simulink model "PMSM_RobotKinematics"  (R2018b)
settings: Solver=VariableStepAuto  StartTime=0.0  StopTime=0.2  FixedStep=Ts  RelTol=1e-4  EnableMultiTasking=on
PreLoadFcn:
  | run('Arm6Assembly_DataFile.m');
model workspace: external: MAT-File E:\SixRobotArm\Simscape_Simulation\StepFile\Arm6Assembly_DataFile.mat (data not in the file)
values from neighbouring files (symbols this model uses):
  smiData =     [Arm6SimscapeData.mat]
undefined symbols (not defined in the file or in its folder): X, Y, Z
libraries: sm_lib x36, fl_lib x25, nesl_utility x19, simulink_extras x7
(part 1 of 4)
settings Model: Creator=SUN  LastModifiedBy=Jeason
settings SolverCC: ZeroCrossControl=DisableAll
settings DataIOCC: LimitDataPoints=on  SaveFormat=Array  SignalLoggingSaveFormat=ModelDataLogs
settings OptimizationCC: ExpressionDepthLimit=2147483647  InitFltsAndDblsToZero=on  LifeSpan=inf
settings DebuggingCC: UnderspecifiedInitializationDetection=Classic  MergeDetectMultiDrivingBlocksExec=none  SolverPrmCheckMsg=warning  FcnCallInpInsideContextMsg=warning  StateNameClashWarn=warning  SFUnexpectedBacktrackingDiag=warning  SFNoUnconditionalDefaultTransitionDiag=warning  SFExecutionAtInitializationDiag=none
settings HardwareCC: ProdBitPerPointer=32  ProdBitPerSizeT=32  ProdBitPerPtrDiffT=32  ProdLargestAtomicFloat=None  ProdIntDivRoundTo=Undefined  ProdEndianess=Unspecified  ProdWordSize=32  ProdHWDeviceType=32-bit Generic
settings ModelReferenceCC: PropagateSignalLabelsOutOfModel=off
settings SFSimCC: SimUseLocalCustomCode=off
settings RTWCC: RTWUseLocalCustomCode=off
settings CodeAppCC: StateflowObjectComments=on
settings GRTTargetCC: TargetLangStandard=C89/C90 (ANSI)  GeneratePreprocessorConditionals=Disable all  CombineOutputUpdateFcns=off  GRTInterface=on
settings ConfigComp: CovMetricSettings=dw  CovHtmlReporting=on  CovSaveCumulativeToWorkspaceVar=on  CovSaveSingleToWorkspaceVar=on  CovExternalEMLEnable=off  CovSFcnEnable=off
settings SimscapeCC: SimscapeNormalizeSystem=off
settings ExplorerConfigSet: InternalSimMechanicsExplorerSettings="<ExplorerConfiguration><canonicalview>planar_xy</canonicalview><AnimationSetting><BasePlaybackSpeed>1.0</BasePlaybackSpeed><PlaybackSpeedFactor>0.015625</PlaybackSpeedFactor></AnimationSetting><TilePanel><TileInfo><Tiles Columns=\"1\" Count=\"1\" Rows=\"1\"><Column Weight=\"1\"/><Row Weight=\"1\"/><Tile Height=\"1\" Width=\"1\" X=\"0\" Y=\"0\"/></Tiles></TileInfo><SceneInfo><SceneViewer><BGColor><R>0.60000002384185791</R><G>0.60000002384185791</G><B>0.60000002384185791</B></BGColor><Camera><DoPerspective>off</DoPerspective><Position><X>0.688113997528940757</X><Y>0.890134013005122293</Y><Z>0.448440006070310149</Z></Position><Center><X>0.110763728339315123</X><Y>0.312783743815496507</Y><Z>-0.128910263119315527</Z></Center><Up><X>-0.408248290463863073</X><Y>0.816496580927726145</Y><Z>-0.408248290463863073</Z></Up><ViewLimDist>1</ViewLimDist><YLim>0.769232078900134564</YLim><XLim>0.559679639699189879</XLim></Camera></SceneViewer></SceneInfo></TilePanel><MechEditorPanel><Cameras/><GfxPanelCameraMap/><VideoCreator><PlaybackSpeedRatio>0.25</PlaybackSpeedRatio><FrameRate>30</FrameRate><VideoFormat>MPEG-4</VideoFormat><FrameSize>auto</FrameSize></VideoCreator></MechEditorPanel></ExplorerConfiguration>"

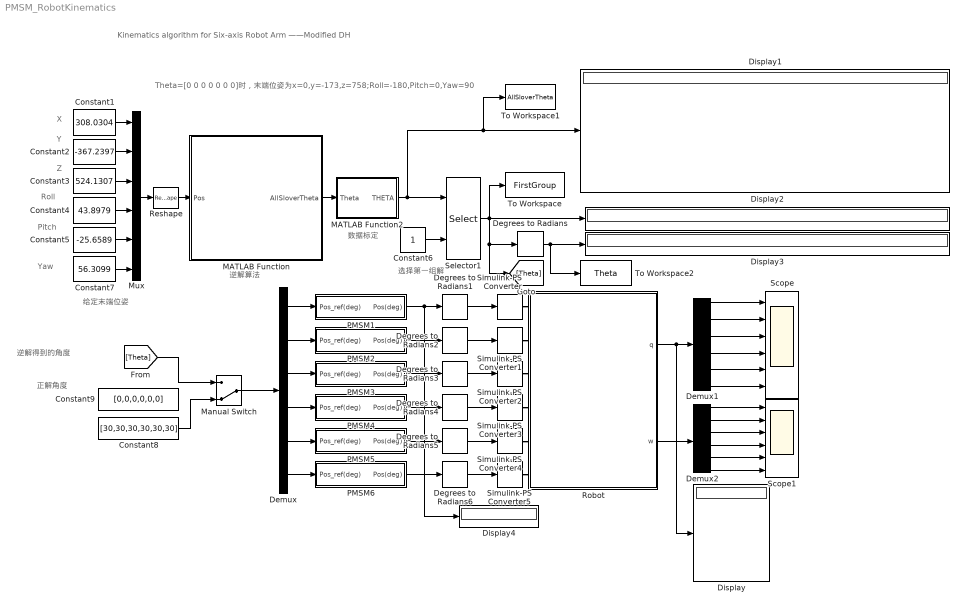
== system PMSM_RobotKinematics ==
  note: 逆解得到的角度
  note: 正解角度
  note: Kinematics algorithm for Six-axis Robot Arm ——Modified DH
  note: X
  note: 选择第一组解
  note: Pitch
  note: Roll
  note: 数据标定
  note: 给定末端位姿
  note: Y
  note: Yaw
  note: Theta=[0 0 0 0 0 0 0]时，末端位姿为x=0,y=-173,z=758;Roll=-180,Pitch=0,Yaw=90
  note: 逆解算法
  note: Z
  Constant1 : Constant  Value=308.0304
  Constant2 : Constant  Value=-367.2397
  Constant3 : Constant  Value=524.1307
  Constant4 : Constant  Value=43.8979
  Constant5 : Constant  Value=-25.6589
  Constant6 : Constant
  Constant7 : Constant  Value=56.3099
  Constant8 : Constant  Value=[30,30,30,30,30,30]
  Constant9 : Constant  Value=[0,0,0,0,0,0]
  Degrees to Radians{,1..6} (7 alike) : simulink_extras/Transformations/Degrees to Radians
  Demux : Demux  Outputs=6
  Demux1 : Demux  Outputs=6
  Demux2 : Demux  Outputs=6
  Display{,1..4} (5 alike) : Display
  MATLAB Function : MATLAB Function  TreatAsAtomicUnit=on
  MATLAB Function2 : MATLAB Function  TreatAsAtomicUnit=on
  Manual Switch : ManualSwitch  CurrentSetting=0
  Mux : Mux  Inputs=6
  PMSM1 : Subsystem
  PMSM2 : Subsystem
  PMSM3 : Subsystem
  PMSM4 : Subsystem
  PMSM5 : Subsystem
  PMSM6 : Subsystem
  Reshape : Reshape  OutputDimensionality=Customize  OutputDimensions=[1,6]
  Robot : Subsystem
  Scope : Scope  NumInputPorts=6
  Scope1 : Scope  NumInputPorts=6
  Selector1 : Selector  NumberOfDimensions=2  InputPortWidth=10  IndexOptions=Index vector (port),Starting index (dialog)  Indices=[1 3],1  OutputSizes=1,6
  Simulink-PS Converter{,1..5} (6 alike) : nesl_utility/Simulink-PS Converter  PhysicalDomain=network_engine_domain  SubClassName=ps_input  LeftPortType=input  RightPortType=output  PseudoPeriodic=off  Frequencies=[]  NoiseDistribution=none  NoiseParameters=[]  Unit=rad  AffineConversion=off  FilteringAndDerivatives=provide  SimscapeFilterOrder=2  InputFilterTimeConstant=-1  UdotUserProvided=0
  To Workspace : ToWorkspace  VariableName=FirstGroup  SampleTime=-1
      settings: MaxDataPoints=1
  To Workspace1 : ToWorkspace  VariableName=AllSloverTheta  SampleTime=-1
      settings: MaxDataPoints=1
  To Workspace2 : ToWorkspace  VariableName=Theta  SampleTime=-1
      settings: MaxDataPoints=1
  wires:
  Demux1/3 -> Scope/3
  Demux2/5 -> Scope1/5
  Constant8/1 -> Manual Switch/2
  Demux/5 -> PMSM5/1(Pos_ref(deg))
  Demux2/4 -> Scope1/4
  Demux1/5 -> Scope/5
  Manual Switch/1 -> Demux/1
  Robot/2(w) -> Demux2/1
  Demux2/3 -> Scope1/3
  Demux1/2 -> Scope/2
  Demux1/6 -> Scope/6
  Demux/4 -> PMSM4/1(Pos_ref(deg))
  Demux2/1 -> Scope1/1
  Demux2/6 -> Scope1/6
  [Theta] -> Manual Switch/1
  Demux/6 -> PMSM6/1(Pos_ref(deg))
  Demux/3 -> PMSM3/1(Pos_ref(deg))
  Demux2/2 -> Scope1/2
  Demux/2 -> PMSM2/1(Pos_ref(deg))
  Demux1/4 -> Scope/4
  Demux/1 -> PMSM1/1(Pos_ref(deg))
  Demux1/1 -> Scope/1
  MATLAB Function2/1(THETA) -> To Workspace1/1, Display1/1, Selector1/1
  MATLAB Function/1(AllSloverTheta) -> MATLAB Function2/1(Theta)
  Constant7/1 -> Mux/6
  Constant4/1 -> Mux/4
  Constant5/1 -> Mux/5
  Constant1/1 -> Mux/1
  Constant3/1 -> Mux/3
  Degrees to Radians/1 -> To Workspace2/1, Display3/1
  Reshape/1 -> MATLAB Function/1(Pos)
  Constant6/1 -> Selector1/2
  Constant2/1 -> Mux/2
  Mux/1 -> Reshape/1
  Selector1/1 -> To Workspace/1, [Theta], Degrees to Radians/1, Display2/1
  PMSM1/1(Pos(deg)) -> Display4/1, Degrees to Radians1/1
  PMSM2/1(Pos(deg)) -> Degrees to Radians2/1
  PMSM3/1(Pos(deg)) -> Degrees to Radians3/1
  PMSM5/1(Pos(deg)) -> Degrees to Radians5/1
  PMSM6/1(Pos(deg)) -> Degrees to Radians6/1
  Robot/1(q) -> Display/1, Demux1/1
  Degrees to Radians1/1 -> Simulink-PS Converter/1
  Degrees to Radians2/1 -> Simulink-PS Converter1/1
  Degrees to Radians3/1 -> Simulink-PS Converter2/1
  Degrees to Radians4/1 -> Simulink-PS Converter3/1
  Degrees to Radians5/1 -> Simulink-PS Converter4/1
  Degrees to Radians6/1 -> Simulink-PS Converter5/1
  PMSM4/1(Pos(deg)) -> Degrees to Radians4/1
  connections:
  Simulink-PS Converter/RConn1 -- Robot/LConn1
  Simulink-PS Converter5/RConn1 -- Robot/LConn6
  Simulink-PS Converter4/RConn1 -- Robot/LConn5
  Simulink-PS Converter3/RConn1 -- Robot/LConn4
  Simulink-PS Converter2/RConn1 -- Robot/LConn3
  Simulink-PS Converter1/RConn1 -- Robot/LConn2

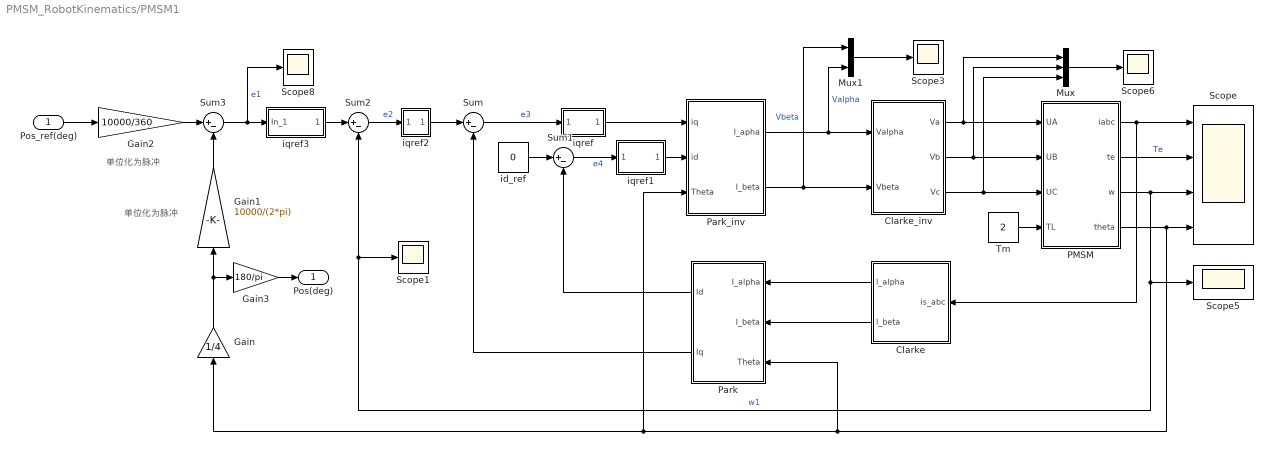
== system PMSM_RobotKinematics/PMSM1 ==
  note: 单位化为脉冲
  note: 单位化为脉冲
  Pos_ref(deg) : Inport
  Clarke : Subsystem
  Clarke_inv : Subsystem
  Gain : Gain  Gain=1/4
  Gain1 : Gain  Gain=10000/(2*pi)
  Gain2 : Gain  Gain=10000/360
  Gain3 : Gain  Gain=180/pi
  Mux : Mux  Inputs=3
  Mux1 : Mux  Inputs=2
  PMSM : Subsystem  mask(hao){CL=0.175, Pm=4, Ld=0.0085, Lq=0.0085, rs=2.875, J=0.0008}
      mask help: pmsm
      mask Help: no
  Park : Subsystem
  Park_inv : Subsystem
  Scope : Scope  NumInputPorts=4
  Scope{1,3,5..6,8} (5 alike) : Scope
  Sum{,1..3} (4 alike) : Sum  Inputs=|+-  SaturateOnIntegerOverflow=on
  Tm : Constant  Value=2
  id_ref : Constant  Value=0
  iqref : Subsystem  mask(PI Controller){I=5, P=10, sat=[-500, 500]}
      mask prompts: I "Integral"; P "Proportional:"; sat "Minimum and maximum outputs:"
      mask init:
      | min=sat(1);max=sat(2);
      mask Display: disp('PI')
  iqref1 : Subsystem  mask(PI Controller){I=5, P=10, sat=[-500, 500]}
      mask prompts: I "Integral"; P "Proportional:"; sat "Minimum and maximum outputs:"
      mask init:
      | min=sat(1);max=sat(2);
      mask Display: disp('PI')
  iqref2 : Subsystem  mask(PI Controller){I=5, P=10, sat=[-30, 30]}
      mask prompts: I "Integral"; P "Proportional:"; sat "Minimum and maximum outputs:"
      mask init:
      | min=sat(1);max=sat(2);
      mask Display: disp('PI')
  iqref3 : Subsystem  mask(PI Controller){I=0.012, P=0.14, sat=[-1000, 1000]}
      mask prompts: I "Integral"; P "Proportional:"; sat "Minimum and maximum outputs:"
      mask init:
      | min=sat(1);max=sat(2);
      mask Display: disp('PI')
  Pos(deg) : Outport
  wires:
  iqref1/1(Out_1) -> Park_inv/2(id)
  Sum3/1 -> Scope8/1, iqref3/1(In_1)  "e1"
  Pos_ref(deg)/1 -> Gain2/1
  Mux1/1 -> Scope3/1
  Sum/1 -> iqref/1(In_1)  "e3"
  PMSM/3(w) -> Scope/3, Sum2/2, Scope1/1, Scope5/1  "w1"
  Tm/1 -> PMSM/4(TL)
  Park/2(Iq) -> Sum/2
  Clarke/1(I_alpha) -> Park/1(I_alpha)
  Clarke_inv/3(Vc) -> PMSM/3(UC), Mux/3
  Park/1(Id) -> Sum1/2
  Mux/1 -> Scope6/1
  Clarke_inv/1(Va) -> PMSM/1(UA), Mux/1
  Sum2/1 -> iqref2/1(In_1)  "e2"
  Park_inv/2(I_beta) -> Mux1/1, Clarke_inv/2(Vbeta)  "Vbeta"
  Gain1/1 -> Sum3/2
  PMSM/4(theta) -> Scope/4, Park/3(Theta), Park_inv/3(Theta), Gain/1
  Clarke_inv/2(Vb) -> PMSM/2(UB), Mux/2
  Gain2/1 -> Sum3/1
  iqref2/1(Out_1) -> Sum/1
  Park_inv/1(I_apha) -> Clarke_inv/1(Valpha), Mux1/2  "Valpha"
  Sum1/1 -> iqref1/1(In_1)  "e4"
  iqref3/1(Out_1) -> Sum2/1
  Clarke/2(I_beta) -> Park/2(I_beta)
  PMSM/2(te) -> Scope/2  "Te"
  iqref/1(Out_1) -> Park_inv/1(iq)
  PMSM/1(iabc) -> Scope/1, Clarke/1(is_abc)
  id_ref/1 -> Sum1/1
  Gain/1 -> Gain1/1, Gain3/1
  Gain3/1 -> Pos(deg)/1

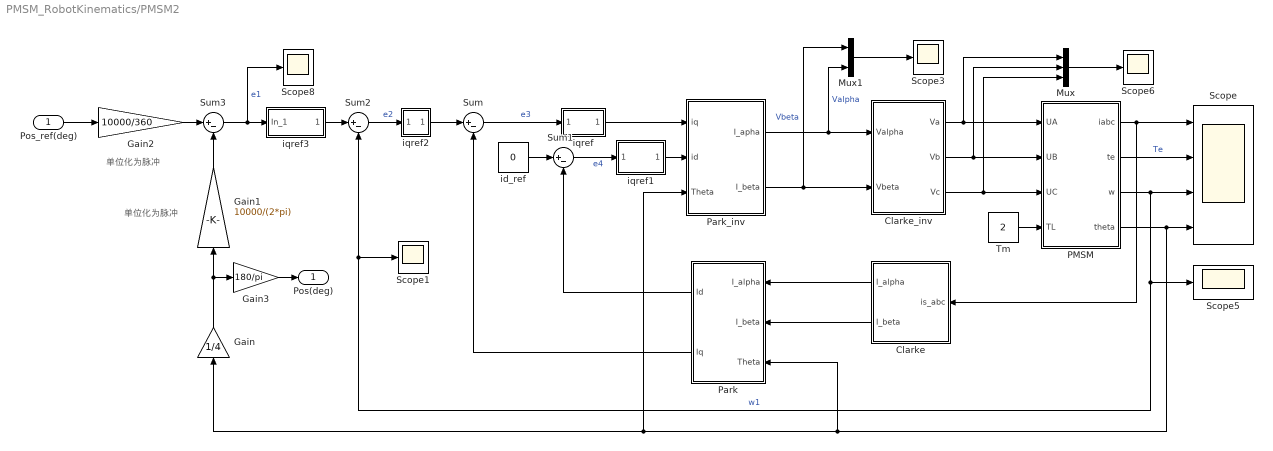
== system PMSM_RobotKinematics/PMSM2 ==
  note: 单位化为脉冲
  note: 单位化为脉冲
  Pos_ref(deg) : Inport
  Clarke : Subsystem
  Clarke_inv : Subsystem
  Gain : Gain  Gain=1/4
  Gain1 : Gain  Gain=10000/(2*pi)
  Gain2 : Gain  Gain=10000/360
  Gain3 : Gain  Gain=180/pi
  Mux : Mux  Inputs=3
  Mux1 : Mux  Inputs=2
  PMSM : Subsystem  mask(hao){CL=0.175, Pm=4, Ld=0.0085, Lq=0.0085, rs=2.875, J=0.0008}
      mask help: pmsm
      mask Help: no
  Park : Subsystem
  Park_inv : Subsystem
  Scope : Scope  NumInputPorts=4
  Scope{1,3,5..6,8} (5 alike) : Scope
  Sum{,1..3} (4 alike) : Sum  Inputs=|+-  SaturateOnIntegerOverflow=on
  Tm : Constant  Value=2
  id_ref : Constant  Value=0
  iqref : Subsystem  mask(PI Controller){I=5, P=10, sat=[-500, 500]}
      mask prompts: I "Integral"; P "Proportional:"; sat "Minimum and maximum outputs:"
      mask init:
      | min=sat(1);max=sat(2);
      mask Display: disp('PI')
  iqref1 : Subsystem  mask(PI Controller){I=5, P=10, sat=[-500, 500]}
      mask prompts: I "Integral"; P "Proportional:"; sat "Minimum and maximum outputs:"
      mask init:
      | min=sat(1);max=sat(2);
      mask Display: disp('PI')
  iqref2 : Subsystem  mask(PI Controller){I=5, P=10, sat=[-30, 30]}
      mask prompts: I "Integral"; P "Proportional:"; sat "Minimum and maximum outputs:"
      mask init:
      | min=sat(1);max=sat(2);
      mask Display: disp('PI')
  iqref3 : Subsystem  mask(PI Controller){I=0.012, P=0.14, sat=[-1000, 1000]}
      mask prompts: I "Integral"; P "Proportional:"; sat "Minimum and maximum outputs:"
      mask init:
      | min=sat(1);max=sat(2);
      mask Display: disp('PI')
  Pos(deg) : Outport
  wires:
  Gain3/1 -> Pos(deg)/1
  Gain/1 -> Gain3/1, Gain1/1
  id_ref/1 -> Sum1/1
  PMSM/1(iabc) -> Clarke/1(is_abc), Scope/1
  iqref/1(Out_1) -> Park_inv/1(iq)
  PMSM/2(te) -> Scope/2  "Te"
  Clarke/2(I_beta) -> Park/2(I_beta)
  iqref3/1(Out_1) -> Sum2/1
  Sum1/1 -> iqref1/1(In_1)  "e4"
  Park_inv/1(I_apha) -> Mux1/2, Clarke_inv/1(Valpha)  "Valpha"
  iqref2/1(Out_1) -> Sum/1
  Gain2/1 -> Sum3/1
  Clarke_inv/2(Vb) -> Mux/2, PMSM/2(UB)
  PMSM/4(theta) -> Gain/1, Park_inv/3(Theta), Park/3(Theta), Scope/4
  Gain1/1 -> Sum3/2
  Park_inv/2(I_beta) -> Clarke_inv/2(Vbeta), Mux1/1  "Vbeta"
  Sum2/1 -> iqref2/1(In_1)  "e2"
  Clarke_inv/1(Va) -> Mux/1, PMSM/1(UA)
  Mux/1 -> Scope6/1
  Park/1(Id) -> Sum1/2
  Clarke_inv/3(Vc) -> Mux/3, PMSM/3(UC)
  Clarke/1(I_alpha) -> Park/1(I_alpha)
  Park/2(Iq) -> Sum/2
  Tm/1 -> PMSM/4(TL)
  PMSM/3(w) -> Scope5/1, Scope1/1, Sum2/2, Scope/3  "w1"
  Sum/1 -> iqref/1(In_1)  "e3"
  Mux1/1 -> Scope3/1
  Pos_ref(deg)/1 -> Gain2/1
  Sum3/1 -> iqref3/1(In_1), Scope8/1  "e1"
  iqref1/1(Out_1) -> Park_inv/2(id)

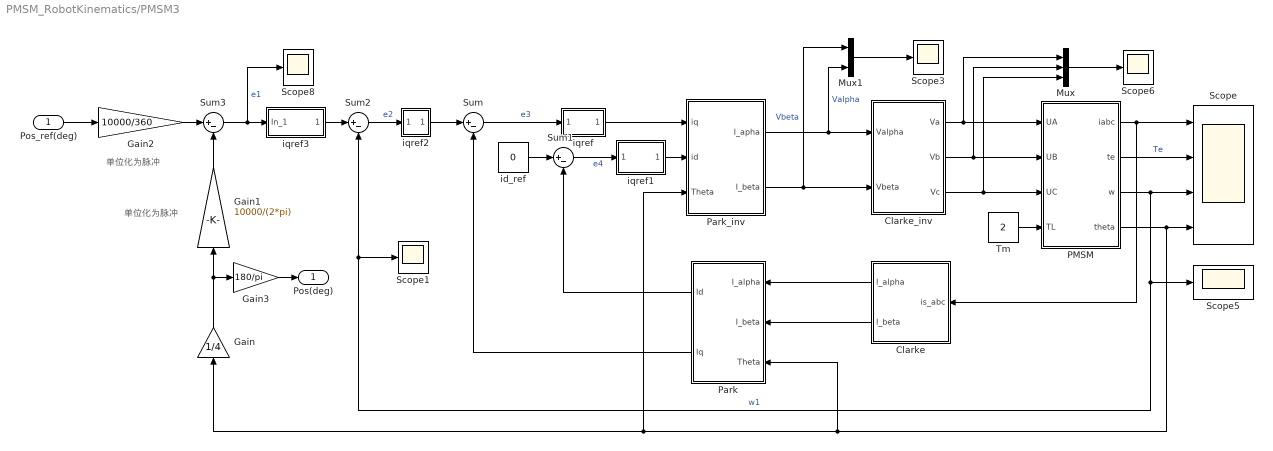
== system PMSM_RobotKinematics/PMSM3 ==
  note: 单位化为脉冲
  note: 单位化为脉冲
  Pos_ref(deg) : Inport
  Clarke : Subsystem
  Clarke_inv : Subsystem
  Gain : Gain  Gain=1/4
  Gain1 : Gain  Gain=10000/(2*pi)
  Gain2 : Gain  Gain=10000/360
  Gain3 : Gain  Gain=180/pi
  Mux : Mux  Inputs=3
  Mux1 : Mux  Inputs=2
  PMSM : Subsystem  mask(hao){CL=0.175, Pm=4, Ld=0.0085, Lq=0.0085, rs=2.875, J=0.0008}
      mask help: pmsm
      mask Help: no
  Park : Subsystem
  Park_inv : Subsystem
  Scope : Scope  NumInputPorts=4
  Scope{1,3,5..6,8} (5 alike) : Scope
  Sum{,1..3} (4 alike) : Sum  Inputs=|+-  SaturateOnIntegerOverflow=on
  Tm : Constant  Value=2
  id_ref : Constant  Value=0
  iqref : Subsystem  mask(PI Controller){I=5, P=10, sat=[-500, 500]}
      mask prompts: I "Integral"; P "Proportional:"; sat "Minimum and maximum outputs:"
      mask init:
      | min=sat(1);max=sat(2);
      mask Display: disp('PI')
  iqref1 : Subsystem  mask(PI Controller){I=5, P=10, sat=[-500, 500]}
      mask prompts: I "Integral"; P "Proportional:"; sat "Minimum and maximum outputs:"
      mask init:
      | min=sat(1);max=sat(2);
      mask Display: disp('PI')
  iqref2 : Subsystem  mask(PI Controller){I=5, P=10, sat=[-30, 30]}
      mask prompts: I "Integral"; P "Proportional:"; sat "Minimum and maximum outputs:"
      mask init:
      | min=sat(1);max=sat(2);
      mask Display: disp('PI')
  iqref3 : Subsystem  mask(PI Controller){I=0.012, P=0.14, sat=[-1000, 1000]}
      mask prompts: I "Integral"; P "Proportional:"; sat "Minimum and maximum outputs:"
      mask init:
      | min=sat(1);max=sat(2);
      mask Display: disp('PI')
  Pos(deg) : Outport
  wires:
  iqref1/1(Out_1) -> Park_inv/2(id)
  Sum3/1 -> Scope8/1, iqref3/1(In_1)  "e1"
  Pos_ref(deg)/1 -> Gain2/1
  Mux1/1 -> Scope3/1
  Sum/1 -> iqref/1(In_1)  "e3"
  PMSM/3(w) -> Scope/3, Sum2/2, Scope1/1, Scope5/1  "w1"
  Tm/1 -> PMSM/4(TL)
  Park/2(Iq) -> Sum/2
  Clarke/1(I_alpha) -> Park/1(I_alpha)
  Clarke_inv/3(Vc) -> PMSM/3(UC), Mux/3
  Park/1(Id) -> Sum1/2
  Mux/1 -> Scope6/1
  Clarke_inv/1(Va) -> PMSM/1(UA), Mux/1
  Sum2/1 -> iqref2/1(In_1)  "e2"
  Park_inv/2(I_beta) -> Mux1/1, Clarke_inv/2(Vbeta)  "Vbeta"
  Gain1/1 -> Sum3/2
  PMSM/4(theta) -> Scope/4, Park/3(Theta), Park_inv/3(Theta), Gain/1
  Clarke_inv/2(Vb) -> PMSM/2(UB), Mux/2
  Gain2/1 -> Sum3/1
  iqref2/1(Out_1) -> Sum/1
  Park_inv/1(I_apha) -> Clarke_inv/1(Valpha), Mux1/2  "Valpha"
  Sum1/1 -> iqref1/1(In_1)  "e4"
  iqref3/1(Out_1) -> Sum2/1
  Clarke/2(I_beta) -> Park/2(I_beta)
  PMSM/2(te) -> Scope/2  "Te"
  iqref/1(Out_1) -> Park_inv/1(iq)
  PMSM/1(iabc) -> Scope/1, Clarke/1(is_abc)
  id_ref/1 -> Sum1/1
  Gain/1 -> Gain1/1, Gain3/1
  Gain3/1 -> Pos(deg)/1

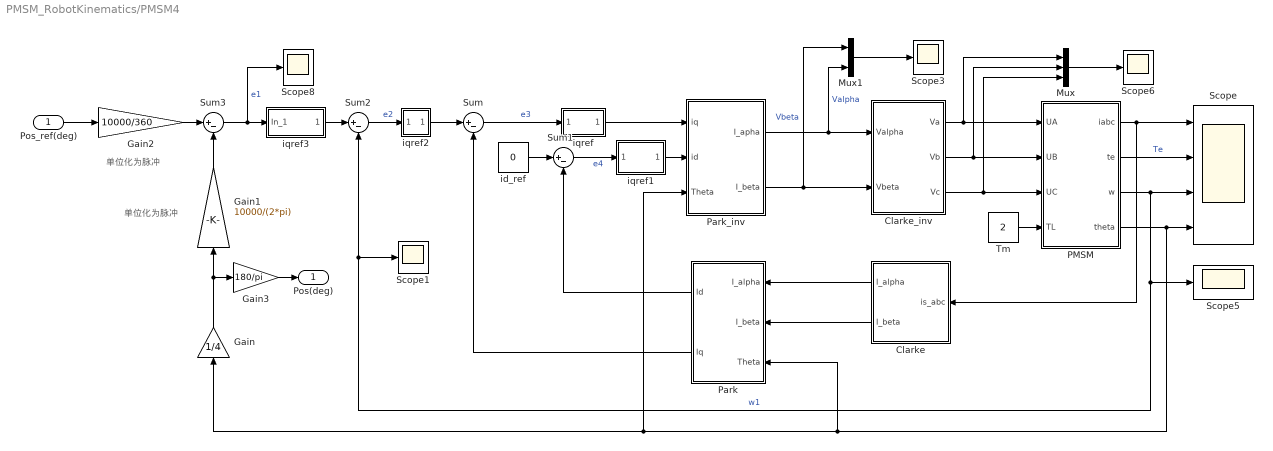
== system PMSM_RobotKinematics/PMSM4 ==
  note: 单位化为脉冲
  note: 单位化为脉冲
  Pos_ref(deg) : Inport
  Clarke : Subsystem
  Clarke_inv : Subsystem
  Gain : Gain  Gain=1/4
  Gain1 : Gain  Gain=10000/(2*pi)
  Gain2 : Gain  Gain=10000/360
  Gain3 : Gain  Gain=180/pi
  Mux : Mux  Inputs=3
  Mux1 : Mux  Inputs=2
  PMSM : Subsystem  mask(hao){CL=0.175, Pm=4, Ld=0.0085, Lq=0.0085, rs=2.875, J=0.0008}
      mask help: pmsm
      mask Help: no
  Park : Subsystem
  Park_inv : Subsystem
  Scope : Scope  NumInputPorts=4
  Scope{1,3,5..6,8} (5 alike) : Scope
  Sum{,1..3} (4 alike) : Sum  Inputs=|+-  SaturateOnIntegerOverflow=on
  Tm : Constant  Value=2
  id_ref : Constant  Value=0
  iqref : Subsystem  mask(PI Controller){I=5, P=10, sat=[-500, 500]}
      mask prompts: I "Integral"; P "Proportional:"; sat "Minimum and maximum outputs:"
      mask init:
      | min=sat(1);max=sat(2);
      mask Display: disp('PI')
  iqref1 : Subsystem  mask(PI Controller){I=5, P=10, sat=[-500, 500]}
      mask prompts: I "Integral"; P "Proportional:"; sat "Minimum and maximum outputs:"
      mask init:
      | min=sat(1);max=sat(2);
      mask Display: disp('PI')
  iqref2 : Subsystem  mask(PI Controller){I=5, P=10, sat=[-30, 30]}
      mask prompts: I "Integral"; P "Proportional:"; sat "Minimum and maximum outputs:"
      mask init:
      | min=sat(1);max=sat(2);
      mask Display: disp('PI')
  iqref3 : Subsystem  mask(PI Controller){I=0.012, P=0.14, sat=[-1000, 1000]}
      mask prompts: I "Integral"; P "Proportional:"; sat "Minimum and maximum outputs:"
      mask init:
      | min=sat(1);max=sat(2);
      mask Display: disp('PI')
  Pos(deg) : Outport
  wires:
  Gain3/1 -> Pos(deg)/1
  Gain/1 -> Gain3/1, Gain1/1
  id_ref/1 -> Sum1/1
  PMSM/1(iabc) -> Clarke/1(is_abc), Scope/1
  iqref/1(Out_1) -> Park_inv/1(iq)
  PMSM/2(te) -> Scope/2  "Te"
  Clarke/2(I_beta) -> Park/2(I_beta)
  iqref3/1(Out_1) -> Sum2/1
  Sum1/1 -> iqref1/1(In_1)  "e4"
  Park_inv/1(I_apha) -> Mux1/2, Clarke_inv/1(Valpha)  "Valpha"
  iqref2/1(Out_1) -> Sum/1
  Gain2/1 -> Sum3/1
  Clarke_inv/2(Vb) -> Mux/2, PMSM/2(UB)
  PMSM/4(theta) -> Gain/1, Park_inv/3(Theta), Park/3(Theta), Scope/4
  Gain1/1 -> Sum3/2
  Park_inv/2(I_beta) -> Clarke_inv/2(Vbeta), Mux1/1  "Vbeta"
  Sum2/1 -> iqref2/1(In_1)  "e2"
  Clarke_inv/1(Va) -> Mux/1, PMSM/1(UA)
  Mux/1 -> Scope6/1
  Park/1(Id) -> Sum1/2
  Clarke_inv/3(Vc) -> Mux/3, PMSM/3(UC)
  Clarke/1(I_alpha) -> Park/1(I_alpha)
  Park/2(Iq) -> Sum/2
  Tm/1 -> PMSM/4(TL)
  PMSM/3(w) -> Scope5/1, Scope1/1, Sum2/2, Scope/3  "w1"
  Sum/1 -> iqref/1(In_1)  "e3"
  Mux1/1 -> Scope3/1
  Pos_ref(deg)/1 -> Gain2/1
  Sum3/1 -> iqref3/1(In_1), Scope8/1  "e1"
  iqref1/1(Out_1) -> Park_inv/2(id)

== system PMSM_RobotKinematics/PMSM5 ==
  note: 单位化为脉冲
  note: 单位化为脉冲
  Pos_ref(deg) : Inport
  Clarke : Subsystem
  Clarke_inv : Subsystem
  Gain : Gain  Gain=1/4
  Gain1 : Gain  Gain=10000/(2*pi)
  Gain2 : Gain  Gain=10000/360
  Gain3 : Gain  Gain=180/pi
  Mux : Mux  Inputs=3
  Mux1 : Mux  Inputs=2
  PMSM : Subsystem  mask(hao){CL=0.175, Pm=4, Ld=0.0085, Lq=0.0085, rs=2.875, J=0.0008}
      mask help: pmsm
      mask Help: no
  Park : Subsystem
  Park_inv : Subsystem
  Scope : Scope  NumInputPorts=4
  Scope{1,3,5..6,8} (5 alike) : Scope
  Sum{,1..3} (4 alike) : Sum  Inputs=|+-  SaturateOnIntegerOverflow=on
  Tm : Constant  Value=2
  id_ref : Constant  Value=0
  iqref : Subsystem  mask(PI Controller){I=5, P=10, sat=[-500, 500]}
      mask prompts: I "Integral"; P "Proportional:"; sat "Minimum and maximum outputs:"
      mask init:
      | min=sat(1);max=sat(2);
      mask Display: disp('PI')
  iqref1 : Subsystem  mask(PI Controller){I=5, P=10, sat=[-500, 500]}
      mask prompts: I "Integral"; P "Proportional:"; sat "Minimum and maximum outputs:"
      mask init:
      | min=sat(1);max=sat(2);
      mask Display: disp('PI')
  iqref2 : Subsystem  mask(PI Controller){I=5, P=10, sat=[-30, 30]}
      mask prompts: I "Integral"; P "Proportional:"; sat "Minimum and maximum outputs:"
      mask init:
      | min=sat(1);max=sat(2);
      mask Display: disp('PI')
  iqref3 : Subsystem  mask(PI Controller){I=0.012, P=0.14, sat=[-1000, 1000]}
      mask prompts: I "Integral"; P "Proportional:"; sat "Minimum and maximum outputs:"
      mask init:
      | min=sat(1);max=sat(2);
      mask Display: disp('PI')
  Pos(deg) : Outport
  wires:
  iqref1/1(Out_1) -> Park_inv/2(id)
  Sum3/1 -> Scope8/1, iqref3/1(In_1)  "e1"
  Pos_ref(deg)/1 -> Gain2/1
  Mux1/1 -> Scope3/1
  Sum/1 -> iqref/1(In_1)  "e3"
  PMSM/3(w) -> Scope/3, Sum2/2, Scope1/1, Scope5/1  "w1"
  Tm/1 -> PMSM/4(TL)
  Park/2(Iq) -> Sum/2
  Clarke/1(I_alpha) -> Park/1(I_alpha)
  Clarke_inv/3(Vc) -> PMSM/3(UC), Mux/3
  Park/1(Id) -> Sum1/2
  Mux/1 -> Scope6/1
  Clarke_inv/1(Va) -> PMSM/1(UA), Mux/1
  Sum2/1 -> iqref2/1(In_1)  "e2"
  Park_inv/2(I_beta) -> Mux1/1, Clarke_inv/2(Vbeta)  "Vbeta"
  Gain1/1 -> Sum3/2
  PMSM/4(theta) -> Scope/4, Park/3(Theta), Park_inv/3(Theta), Gain/1
  Clarke_inv/2(Vb) -> PMSM/2(UB), Mux/2
  Gain2/1 -> Sum3/1
  iqref2/1(Out_1) -> Sum/1
  Park_inv/1(I_apha) -> Clarke_inv/1(Valpha), Mux1/2  "Valpha"
  Sum1/1 -> iqref1/1(In_1)  "e4"
  iqref3/1(Out_1) -> Sum2/1
  Clarke/2(I_beta) -> Park/2(I_beta)
  PMSM/2(te) -> Scope/2  "Te"
  iqref/1(Out_1) -> Park_inv/1(iq)
  PMSM/1(iabc) -> Scope/1, Clarke/1(is_abc)
  id_ref/1 -> Sum1/1
  Gain/1 -> Gain1/1, Gain3/1
  Gain3/1 -> Pos(deg)/1

== system PMSM_RobotKinematics/PMSM6 ==
  note: 单位化为脉冲
  note: 单位化为脉冲
  Pos_ref(deg) : Inport
  Clarke : Subsystem
  Clarke_inv : Subsystem
  Gain : Gain  Gain=1/4
  Gain1 : Gain  Gain=10000/(2*pi)
  Gain2 : Gain  Gain=10000/360
  Gain3 : Gain  Gain=180/pi
  Mux : Mux  Inputs=3
  Mux1 : Mux  Inputs=2
  PMSM : Subsystem  mask(hao){CL=0.175, Pm=4, Ld=0.0085, Lq=0.0085, rs=2.875, J=0.0008}
      mask help: pmsm
      mask Help: no
  Park : Subsystem
  Park_inv : Subsystem
  Scope : Scope  NumInputPorts=4
  Scope{1,3,5..6,8} (5 alike) : Scope
  Sum{,1..3} (4 alike) : Sum  Inputs=|+-  SaturateOnIntegerOverflow=on
  Tm : Constant  Value=2
  id_ref : Constant  Value=0
  iqref : Subsystem  mask(PI Controller){I=5, P=10, sat=[-500, 500]}
      mask prompts: I "Integral"; P "Proportional:"; sat "Minimum and maximum outputs:"
      mask init:
      | min=sat(1);max=sat(2);
      mask Display: disp('PI')
  iqref1 : Subsystem  mask(PI Controller){I=5, P=10, sat=[-500, 500]}
      mask prompts: I "Integral"; P "Proportional:"; sat "Minimum and maximum outputs:"
      mask init:
      | min=sat(1);max=sat(2);
      mask Display: disp('PI')
  iqref2 : Subsystem  mask(PI Controller){I=5, P=10, sat=[-30, 30]}
      mask prompts: I "Integral"; P "Proportional:"; sat "Minimum and maximum outputs:"
      mask init:
      | min=sat(1);max=sat(2);
      mask Display: disp('PI')
  iqref3 : Subsystem  mask(PI Controller){I=0.012, P=0.14, sat=[-1000, 1000]}
      mask prompts: I "Integral"; P "Proportional:"; sat "Minimum and maximum outputs:"
      mask init:
      | min=sat(1);max=sat(2);
      mask Display: disp('PI')
  Pos(deg) : Outport
  wires:
  Gain3/1 -> Pos(deg)/1
  Gain/1 -> Gain3/1, Gain1/1
  id_ref/1 -> Sum1/1
  PMSM/1(iabc) -> Clarke/1(is_abc), Scope/1
  iqref/1(Out_1) -> Park_inv/1(iq)
  PMSM/2(te) -> Scope/2  "Te"
  Clarke/2(I_beta) -> Park/2(I_beta)
  iqref3/1(Out_1) -> Sum2/1
  Sum1/1 -> iqref1/1(In_1)  "e4"
  Park_inv/1(I_apha) -> Mux1/2, Clarke_inv/1(Valpha)  "Valpha"
  iqref2/1(Out_1) -> Sum/1
  Gain2/1 -> Sum3/1
  Clarke_inv/2(Vb) -> Mux/2, PMSM/2(UB)
  PMSM/4(theta) -> Gain/1, Park_inv/3(Theta), Park/3(Theta), Scope/4
  Gain1/1 -> Sum3/2
  Park_inv/2(I_beta) -> Clarke_inv/2(Vbeta), Mux1/1  "Vbeta"
  Sum2/1 -> iqref2/1(In_1)  "e2"
  Clarke_inv/1(Va) -> Mux/1, PMSM/1(UA)
  Mux/1 -> Scope6/1
  Park/1(Id) -> Sum1/2
  Clarke_inv/3(Vc) -> Mux/3, PMSM/3(UC)
  Clarke/1(I_alpha) -> Park/1(I_alpha)
  Park/2(Iq) -> Sum/2
  Tm/1 -> PMSM/4(TL)
  PMSM/3(w) -> Scope5/1, Scope1/1, Sum2/2, Scope/3  "w1"
  Sum/1 -> iqref/1(In_1)  "e3"
  Mux1/1 -> Scope3/1
  Pos_ref(deg)/1 -> Gain2/1
  Sum3/1 -> iqref3/1(In_1), Scope8/1  "e1"
  iqref1/1(Out_1) -> Park_inv/2(id)

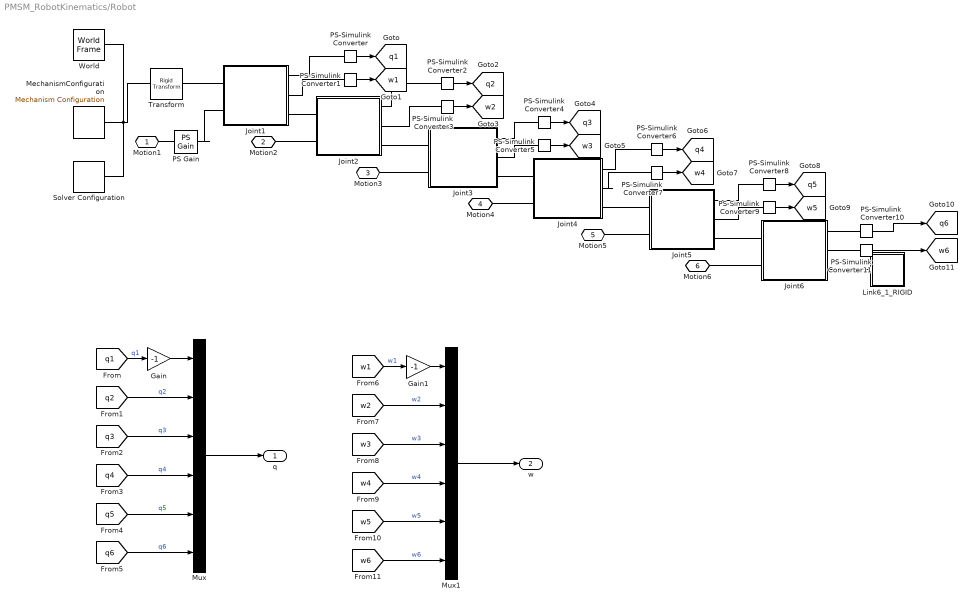
== system PMSM_RobotKinematics/Robot ==
  Gain : Gain  Gain=-1
  Gain1 : Gain  Gain=-1
  Joint1 : Subsystem
  Joint2 : Subsystem
  Joint3 : Subsystem
  Joint4 : Subsystem
  Joint5 : Subsystem
  Joint6 : Subsystem
  Link6_1_RIGID : Subsystem
  MechanismConfiguration : sm_lib/Utilities/Mechanism Configuration  UniformGravity=Constant  GravityVector=[0 -9.80665 0]  GravityUnits=m/s^2  LinearizationDelta=0.001
  Mux : Mux  Inputs=6
  Mux1 : Mux  Inputs=6
  PS Gain : fl_lib/Physical Signals/Functions/PS Gain  gain=-1
  PS-Simulink Converter{,2,4,6,8,10} (6 alike) : nesl_utility/PS-Simulink Converter  PhysicalDomain=network_engine_domain  SubClassName=ps_output  LeftPortType=input  RightPortType=output  PseudoPeriodic=off  Frequencies=[]  Unit=deg  AffineConversion=off
  PS-Simulink Converter{1,3,5,7,9,11} (6 alike) : nesl_utility/PS-Simulink Converter  PhysicalDomain=network_engine_domain  SubClassName=ps_output  LeftPortType=input  RightPortType=output  PseudoPeriodic=off  Frequencies=[]  Unit=deg/s  AffineConversion=off
  Solver Configuration : nesl_utility/Solver Configuration  PhysicalDomain=network_engine_domain  SubClassName=solver  LeftPortType=input  RightPortType=generic  Tones=[]  Harmonics=[]  SimulateNoise=off  Profile=off  UseLocalSampling=off  EnableSwitchedLinearOptims=on  FrequencyDomain=off  UseCCode=off  RelTol=0.001  AbsTol=1e-06  MinStep=1e-09  ToWorkspace=off  RevertToSquareIcSolve=off  NumHomotopyIterations=100  PhasorMode=off  PhasorModeNumHarmonics=1  DoDC=off  ResidualTolerance=1e-09  UseLocalSolver=off  LocalSolverChoice=NE_BACKWARD_EULER_ADVANCER  LocalSolverSampleTime=0.001  DoFixedCost=off  MaxNonlinIter=3  MaxModeIter=2  LinearAlgebra=auto  EquationFormulation=NE_TIME_EF  DelaysMemoryBudget=1024  AutomaticFiltering=on  FilteringTimeConstant=0.001  PartitionStorageMethod=AS_NEEDED  PartitionMemoryBudget=1024
  Transform : sm_lib/Frames and Transforms/Rigid Transform  TranslationMethod=Cartesian  TranslationStandardOffset=0  TranslationLengthUnit=mm  TranslationStandardAxis=+Z  TranslationCartesianOffset=smiData.RigidTransform(14).translation  TranslationROffset=0  TranslationROffsetUnits=m  TranslationZOffset=0  TranslationZOffsetUnits=m  TranslationThetaOffset=0  TranslationThetaOffsetUnits=deg  RotationMethod=ArbitraryAxis  RotationAngleUnits=rad  RotationStandardAxis=+Z  RotationAngle=smiData.RigidTransform(14).angle  RotationArbitraryAxis=smiData.RigidTransform(14).axis  FollAlignAxisA=+X  BaseAlignAxisA=+Y  FollAlignAxisB=+Y  BaseAlignAxisB=+Z  RotationSequenceAxes=FollowerAxes  RotationSequence=XYX  RotationSequenceAngles=[0 0 0]  RotationSequenceAnglesUnits=deg  RotationMatrix=[1 0 0; 0 1 0; 0 0 1]
  World : sm_lib/Frames and Transforms/World Frame
  Motion1 : PMIOPort  Side=Left
  Motion2 : PMIOPort  Port=2  Side=Left
  Motion3 : PMIOPort  Port=3  Side=Left
  Motion4 : PMIOPort  Port=4  Side=Left
  Motion5 : PMIOPort  Port=5  Side=Left
  Motion6 : PMIOPort  Port=6  Side=Left
  q : Outport  VectorParamsAs1DForOutWhenUnconnected=on
  w : Outport  Port=2  VectorParamsAs1DForOutWhenUnconnected=on
  tag scope: q1=global, q2=global, q3=global, q4=global, q5=global, q6=global, w1=global, w2=global, w3=global, w4=global, w5=global, w6=global
  wires:
  [q5] -> Mux/5  "q5"
  Mux/1 -> q/1
  PS-Simulink Converter6/1 -> [q4]
  [w4] -> Mux1/4  "w4"
  PS-Simulink Converter/1 -> [q1]
  [q6] -> Mux/6  "q6"
  [w1] -> Gain1/1  "w1"
  [w5] -> Mux1/5  "w5"
  PS-Simulink Converter4/1 -> [q3]
  PS-Simulink Converter5/1 -> [w3]
  PS-Simulink Converter9/1 -> [w5]
  [w2] -> Mux1/2  "w2"
  PS-Simulink Converter1/1 -> [w1]
  [q2] -> Mux/2  "q2"
  PS-Simulink Converter10/1 -> [q6]
  [w6] -> Mux1/6  "w6"
  PS-Simulink Converter7/1 -> [w4]
  [q4] -> Mux/4  "q4"
  PS-Simulink Converter11/1 -> [w6]
  PS-Simulink Converter8/1 -> [q5]
  Mux1/1 -> w/1
  PS-Simulink Converter2/1 -> [q2]
  [q3] -> Mux/3  "q3"
  [q1] -> Gain/1  "q1"
  [w3] -> Mux1/3  "w3"
  PS-Simulink Converter3/1 -> [w2]
  Gain/1 -> Mux/1
  Gain1/1 -> Mux1/1
  connections:
  Joint6/RConn1 -- PS-Simulink Converter10/LConn1
  PS-Simulink Converter11/LConn1 -- Joint6/RConn2
  Joint4/RConn2 -- PS-Simulink Converter7/LConn1
  Joint4/RConn1 -- PS-Simulink Converter6/LConn1
  PS-Simulink Converter9/LConn1 -- Joint5/RConn2
  PS-Simulink Converter5/LConn1 -- Joint3/RConn2
  Transform/LConn1 -- MechanismConfiguration/RConn1 -- Solver Configuration/RConn1 -- World/RConn1
  Joint3/RConn3 -- Joint4/LConn1
  Joint1/RConn2 -- PS-Simulink Converter1/LConn1
  PS-Simulink Converter3/LConn1 -- Joint2/RConn2
  Joint1/LConn1 -- Transform/RConn1
  PS-Simulink Converter8/LConn1 -- Joint5/RConn1
  Motion4/RConn1 -- Joint4/LConn2
  PS-Simulink Converter4/LConn1 -- Joint3/RConn1
  Joint1/RConn1 -- PS-Simulink Converter/LConn1
  Joint6/LConn1 -- Joint5/RConn3
  Joint3/LConn1 -- Joint2/RConn3
  Joint5/LConn1 -- Joint4/RConn3
  Link6_1_RIGID/LConn1 -- Joint6/RConn3
  Motion6/RConn1 -- Joint6/LConn2
  Motion2/RConn1 -- Joint2/LConn2
  PS-Simulink Converter2/LConn1 -- Joint2/RConn1
  Motion5/RConn1 -- Joint5/LConn2
  Joint2/LConn1 -- Joint1/RConn3
  Motion3/RConn1 -- Joint3/LConn2
  PS Gain/RConn1 -- Joint1/LConn2
  Motion1/RConn1 -- PS Gain/LConn1

== system PMSM_RobotKinematics/PMSM1/Clarke ==
  is_abc : Inport
  Gain : Gain  Gain=sqrt(3/2)  SaturateOnIntegerOverflow=on  OutDataTypeStr=Inherit: Same as input  ParamDataTypeStr=Inherit: Same as input
  Gain1 : Gain  Gain=sqrt(2)/2  SaturateOnIntegerOverflow=on  OutDataTypeStr=Inherit: Same as input  ParamDataTypeStr=Inherit: Same as input
  Mux : Mux  Inputs=[3]
  i_alpha : Fcn  Expr=u[1]
  i_beta : Fcn  Expr=u[1]+2*u[2]
  I_alpha : Outport  InitialOutput=0
  I_beta : Outport  Port=2  InitialOutput=0
  wires:
  Mux/1 -> i_beta/1, i_alpha/1
  is_abc/1 -> Mux/1
  i_beta/1 -> Gain1/1
  i_alpha/1 -> Gain/1
  Gain/1 -> I_alpha/1
  Gain1/1 -> I_beta/1

== system PMSM_RobotKinematics/PMSM1/Clarke_inv ==
  Valpha : Inport
  Vbeta : Inport  Port=2
  Fcn : Fcn  Expr=-u[1]/2+1.73205081*u[2]/2
  Fcn1 : Fcn  Expr=-u[1]/2-1.73205081*u[2]/2
  Gain1 : Gain  Gain=sqrt(2/3)  SaturateOnIntegerOverflow=on  OutDataTypeStr=Inherit: Same as input  ParamDataTypeStr=Inherit: Same as input
  Gain2 : Gain  Gain=sqrt(2/3)  SaturateOnIntegerOverflow=on  OutDataTypeStr=Inherit: Same as input  ParamDataTypeStr=Inherit: Same as input
  Gain3 : Gain  Gain=sqrt(2/3)  SaturateOnIntegerOverflow=on  OutDataTypeStr=Inherit: Same as input  ParamDataTypeStr=Inherit: Same as input
  Mux : Mux  Inputs=2
  Va : Outport
  Vb : Outport  Port=2
  Vc : Outport  Port=3
  wires:
  Mux/1 -> Fcn/1, Fcn1/1
  Fcn/1 -> Gain2/1
  Fcn1/1 -> Gain3/1
  Valpha/1 -> Mux/1, Gain1/1
  Vbeta/1 -> Mux/2
  Gain1/1 -> Va/1
  Gain2/1 -> Vb/1
  Gain3/1 -> Vc/1

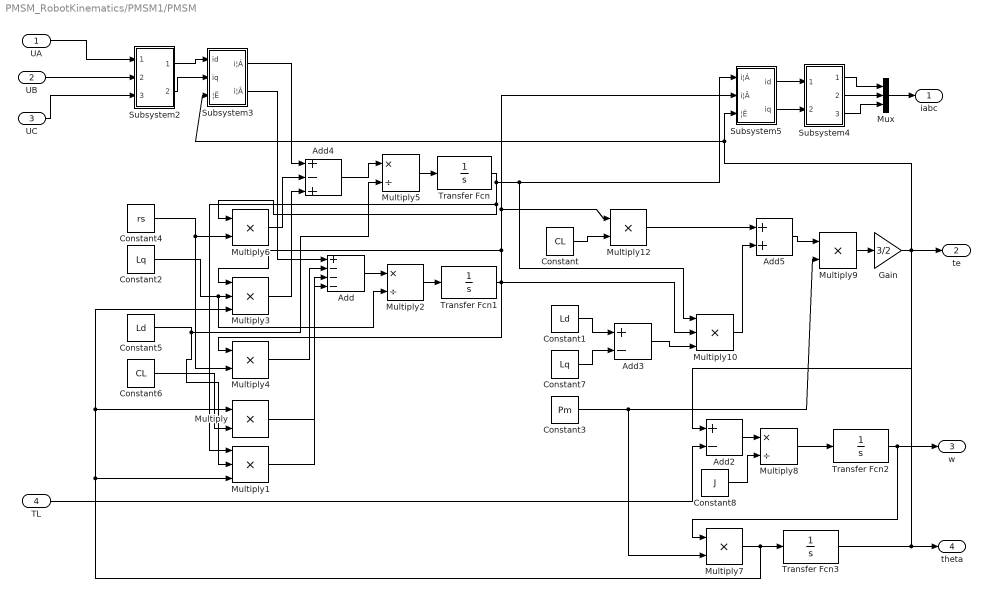
== system PMSM_RobotKinematics/PMSM1/PMSM ==
  UA : Inport
  UB : Inport  Port=2
  UC : Inport  Port=3
  TL : Inport  Port=4
  Add : Sum  Inputs=+---  SaturateOnIntegerOverflow=on  OutDataTypeStr=Inherit: Same as first input
  Add2 : Sum  Inputs=+-  SaturateOnIntegerOverflow=on  InputSameDT=on  OutDataTypeStr=Inherit: Same as first input
  Add3 : Sum  Inputs=+-  SaturateOnIntegerOverflow=on  InputSameDT=on  OutDataTypeStr=Inherit: Same as first input
  Add4 : Sum  Inputs=+-+  SaturateOnIntegerOverflow=on  InputSameDT=on  OutDataTypeStr=Inherit: Same as first input
  Add5 : Sum  SaturateOnIntegerOverflow=on  InputSameDT=on  OutDataTypeStr=Inherit: Same as first input
  Constant : Constant  Value=CL
  Constant1 : Constant  Value=Ld
  Constant2 : Constant  Value=Lq
  Constant3 : Constant  Value=Pm
  Constant4 : Constant  Value=rs
  Constant5 : Constant  Value=Ld
  Constant6 : Constant  Value=CL
  Constant7 : Constant  Value=Lq
  Constant8 : Constant  Value=J
  Gain : Gain  Gain=3/2  SaturateOnIntegerOverflow=on  OutDataTypeStr=Inherit: Same as input  ParamDataTypeStr=Inherit: Same as input
  Multiply{,4,6..7,9,12} (6 alike) : Product  Inputs=**  SaturateOnIntegerOverflow=on  OutDataTypeStr=Inherit: Same as first input
  Multiply1 : Product  Inputs=***  SaturateOnIntegerOverflow=on  OutDataTypeStr=Inherit: Same as first input
  Multiply10 : Product  Inputs=***  SaturateOnIntegerOverflow=on  OutDataTypeStr=Inherit: Same as first input
  Multiply2 : Product  Inputs=*/  SaturateOnIntegerOverflow=on  OutDataTypeStr=Inherit: Same as first input
  Multiply3 : Product  Inputs=***  SaturateOnIntegerOverflow=on  OutDataTypeStr=Inherit: Same as first input
  Multiply5 : Product  Inputs=*/  SaturateOnIntegerOverflow=on  OutDataTypeStr=Inherit: Same as first input
  Multiply8 : Product  Inputs=*/  SaturateOnIntegerOverflow=on  OutDataTypeStr=Inherit: Same as first input
  Mux : Mux  Inputs=3
  Subsystem2 : Subsystem  mask(hao){}
      mask help: 3/2
      mask Help: no
      mask Display: disp('3/2')
  Subsystem3 : Subsystem  mask(2/2){}
      mask help: qdtoMT
      mask Help: none
  Subsystem4 : Subsystem  mask(hao){}
      mask help: 2/3
      mask Help: npi
      mask Display: disp('2/3')
  Subsystem5 : Subsystem  mask(2/2){}
      mask help: mt-todq
      mask Help: no
  Transfer Fcn : TransferFcn  Denominator=[1 0]  AbsoluteTolerance=1e-3
  Transfer Fcn1 : TransferFcn  Denominator=[1 0]
  Transfer Fcn2 : TransferFcn  Denominator=[1 0]
  Transfer Fcn3 : TransferFcn  Denominator=[1 0]
  iabc : Outport
  te : Outport  Port=2
  w : Outport  Port=3
  theta : Outport  Port=4
  wires:
  Multiply2/1 -> Transfer Fcn1/1
  Multiply5/1 -> Transfer Fcn/1
  TL/1 -> Add2/2
  Constant8/1 -> Multiply8/2
  Add2/1 -> Multiply8/1
  Subsystem5/2(iq) -> Subsystem4/2(In3)
  Subsystem5/1(id) -> Subsystem4/1(In1)
  Constant3/1 -> Multiply7/2, Multiply9/2
  Multiply10/1 -> Add5/2
  Multiply12/1 -> Add5/1
  Constant7/1 -> Add3/2
  Constant1/1 -> Add3/1
  Multiply1/1 -> Add/4
  Multiply/1 -> Add/3
  Multiply4/1 -> Add/2
  Add/1 -> Multiply2/1
  Subsystem3/2(i¦Â) -> Add/1
  Add4/1 -> Multiply5/1
  Multiply3/1 -> Add4/3
  Multiply6/1 -> Add4/2
  Subsystem3/1(i¦Á) -> Add4/1
  Subsystem2/2(Out2) -> Subsystem3/2(iq)
  Subsystem2/1(Out1) -> Subsystem3/1(id)
  Transfer Fcn/1 -> Multiply6/1, Multiply1/1, Multiply10/1, Subsystem5/1(i¦Á)
  Constant4/1 -> Multiply6/2, Multiply4/2
  Transfer Fcn1/1 -> Multiply3/1, Multiply12/1, Subsystem5/2(i¦Â), Multiply4/1, Multiply10/2
  Constant2/1 -> Multiply3/2, Multiply2/2
  Constant5/1 -> Multiply1/2, Multiply5/2
  Constant6/1 -> Multiply/2
  Multiply7/1 -> Transfer Fcn3/1, Multiply3/3, Multiply/1, Multiply1/3
  Constant/1 -> Multiply12/2
  Add3/1 -> Multiply10/3
  Transfer Fcn2/1 -> Multiply7/1, w/1
  Add5/1 -> Multiply9/1
  Multiply9/1 -> Gain/1
  Subsystem4/3(Out3) -> Mux/3
  Mux/1 -> iabc/1
  Multiply8/1 -> Transfer Fcn2/1
  UC/1 -> Subsystem2/3(In3)
  Transfer Fcn3/1 -> Subsystem5/3(¦Ë), Subsystem3/3(¦Ë), theta/1
  Gain/1 -> te/1, Add2/1
  Subsystem4/1(Out1) -> Mux/1
  Subsystem4/2(Out2) -> Mux/2
  UA/1 -> Subsystem2/1(In1)
  UB/1 -> Subsystem2/2(In2)

== system PMSM_RobotKinematics/PMSM1/Park ==
  I_alpha : Inport
  I_beta : Inport  Port=2
  Theta : Inport  Port=3
  Fcn : Fcn  Expr=sin(u)
  Fcn1 : Fcn  Expr=cos(u)
  Gain : Gain  SaturateOnIntegerOverflow=on  OutDataTypeStr=Inherit: Same as input  ParamDataTypeStr=Inherit: Same as input
  Gain1 : Gain  SaturateOnIntegerOverflow=on  OutDataTypeStr=Inherit: Same as input  ParamDataTypeStr=Inherit: Same as input
  Mux : Mux  Inputs=[1 1 1 1]
  id : Fcn  Expr=u[1]*u[3]+u[2]*u[4]
  iq : Fcn  Expr=-u[2]*u[3]+u[1]*u[4]
  Id : Outport  InitialOutput=0
  Iq : Outport  Port=2  InitialOutput=0
  wires:
  Fcn/1 -> Mux/2
  Fcn1/1 -> Mux/1
  Theta/1 -> Fcn1/1, Fcn/1
  Mux/1 -> iq/1, id/1
  I_alpha/1 -> Mux/3
  iq/1 -> Gain1/1
  id/1 -> Gain/1
  Gain/1 -> Id/1
  Gain1/1 -> Iq/1
  I_beta/1 -> Mux/4

== system PMSM_RobotKinematics/PMSM1/Park_inv ==
  iq : Inport
  id : Inport  Port=2
  Theta : Inport  Port=3
  Fcn : Fcn  Expr=sin(u)
  Fcn1 : Fcn  Expr=cos(u)
  Gain : Gain  SaturateOnIntegerOverflow=on  OutDataTypeStr=Inherit: Same as input  ParamDataTypeStr=Inherit: Same as input
  Gain1 : Gain  SaturateOnIntegerOverflow=on  OutDataTypeStr=Inherit: Same as input  ParamDataTypeStr=Inherit: Same as input
  Mux : Mux  Inputs=[1 1 1 1]
  i_alpha : Fcn  Expr=u[1]*u[4]-u[2]*u[3]
  i_beta : Fcn  Expr=u[2]*u[4]+u[1]*u[3]
  I_apha : Outport  InitialOutput=0
  I_beta : Outport  Port=2  InitialOutput=0
  wires:
  Fcn/1 -> Mux/2
  Fcn1/1 -> Mux/1
  Theta/1 -> Fcn1/1, Fcn/1
  Mux/1 -> i_beta/1, i_alpha/1
  iq/1 -> Mux/3
  i_beta/1 -> Gain1/1
  i_alpha/1 -> Gain/1
  Gain/1 -> I_apha/1
  Gain1/1 -> I_beta/1
  id/1 -> Mux/4

== system PMSM_RobotKinematics/PMSM1/iqref ==
  In_1 : Inport
  Integral : TransferFcn  Numerator=[I]  Denominator=[1 0]
  Proportional : Gain  Gain=P  SaturateOnIntegerOverflow=on  OutDataTypeStr=Inherit: Same as input  ParamDataTypeStr=Inherit: Same as input
  Saturation : Saturate  UpperLimit=max  LowerLimit=min
  Sum : Sum  SaturateOnIntegerOverflow=on  InputSameDT=on  OutDataTypeStr=Inherit: Same as first input
  Out_1 : Outport  InitialOutput=0
  wires:
  Integral/1 -> Sum/2
  In_1/1 -> Integral/1, Proportional/1
  Proportional/1 -> Sum/1
  Sum/1 -> Saturation/1
  Saturation/1 -> Out_1/1

== system PMSM_RobotKinematics/PMSM1/iqref1 ==
  In_1 : Inport
  Integral : TransferFcn  Numerator=[I]  Denominator=[1 0]
  Proportional : Gain  Gain=P  SaturateOnIntegerOverflow=on  OutDataTypeStr=Inherit: Same as input  ParamDataTypeStr=Inherit: Same as input
  Saturation : Saturate  UpperLimit=max  LowerLimit=min
  Sum : Sum  SaturateOnIntegerOverflow=on  InputSameDT=on  OutDataTypeStr=Inherit: Same as first input
  Out_1 : Outport  InitialOutput=0
  wires:
  Saturation/1 -> Out_1/1
  Sum/1 -> Saturation/1
  Proportional/1 -> Sum/1
  In_1/1 -> Proportional/1, Integral/1
  Integral/1 -> Sum/2

== system PMSM_RobotKinematics/PMSM1/iqref2 ==
  In_1 : Inport
  Integral : TransferFcn  Numerator=[I]  Denominator=[1 0]
  Proportional : Gain  Gain=P  SaturateOnIntegerOverflow=on  OutDataTypeStr=Inherit: Same as input  ParamDataTypeStr=Inherit: Same as input
  Saturation : Saturate  UpperLimit=max  LowerLimit=min
  Sum : Sum  SaturateOnIntegerOverflow=on  InputSameDT=on  OutDataTypeStr=Inherit: Same as first input
  Out_1 : Outport  InitialOutput=0
  wires:
  Saturation/1 -> Out_1/1
  Sum/1 -> Saturation/1
  Proportional/1 -> Sum/1
  In_1/1 -> Proportional/1, Integral/1
  Integral/1 -> Sum/2

== system PMSM_RobotKinematics/PMSM1/iqref3 ==
  In_1 : Inport
  Integral : TransferFcn  Numerator=[I]  Denominator=[1 0]
  Proportional : Gain  Gain=P  SaturateOnIntegerOverflow=on  OutDataTypeStr=Inherit: Same as input  ParamDataTypeStr=Inherit: Same as input
  Saturation : Saturate  UpperLimit=max  LowerLimit=min
  Sum : Sum  SaturateOnIntegerOverflow=on  InputSameDT=on  OutDataTypeStr=Inherit: Same as first input
  Out_1 : Outport  InitialOutput=0
  wires:
  Integral/1 -> Sum/2
  In_1/1 -> Integral/1, Proportional/1
  Proportional/1 -> Sum/1
  Sum/1 -> Saturation/1
  Saturation/1 -> Out_1/1

== system PMSM_RobotKinematics/PMSM2/Clarke ==
  is_abc : Inport
  Gain : Gain  Gain=sqrt(3/2)  SaturateOnIntegerOverflow=on  OutDataTypeStr=Inherit: Same as input  ParamDataTypeStr=Inherit: Same as input
  Gain1 : Gain  Gain=sqrt(2)/2  SaturateOnIntegerOverflow=on  OutDataTypeStr=Inherit: Same as input  ParamDataTypeStr=Inherit: Same as input
  Mux : Mux  Inputs=[3]
  i_alpha : Fcn  Expr=u[1]
  i_beta : Fcn  Expr=u[1]+2*u[2]
  I_alpha : Outport  InitialOutput=0
  I_beta : Outport  Port=2  InitialOutput=0
  wires:
  Gain1/1 -> I_beta/1
  Gain/1 -> I_alpha/1
  i_alpha/1 -> Gain/1
  i_beta/1 -> Gain1/1
  is_abc/1 -> Mux/1
  Mux/1 -> i_alpha/1, i_beta/1

== system PMSM_RobotKinematics/PMSM2/Clarke_inv ==
  Valpha : Inport
  Vbeta : Inport  Port=2
  Fcn : Fcn  Expr=-u[1]/2+1.73205081*u[2]/2
  Fcn1 : Fcn  Expr=-u[1]/2-1.73205081*u[2]/2
  Gain1 : Gain  Gain=sqrt(2/3)  SaturateOnIntegerOverflow=on  OutDataTypeStr=Inherit: Same as input  ParamDataTypeStr=Inherit: Same as input
  Gain2 : Gain  Gain=sqrt(2/3)  SaturateOnIntegerOverflow=on  OutDataTypeStr=Inherit: Same as input  ParamDataTypeStr=Inherit: Same as input
  Gain3 : Gain  Gain=sqrt(2/3)  SaturateOnIntegerOverflow=on  OutDataTypeStr=Inherit: Same as input  ParamDataTypeStr=Inherit: Same as input
  Mux : Mux  Inputs=2
  Va : Outport
  Vb : Outport  Port=2
  Vc : Outport  Port=3
  wires:
  Gain3/1 -> Vc/1
  Gain2/1 -> Vb/1
  Gain1/1 -> Va/1
  Vbeta/1 -> Mux/2
  Valpha/1 -> Gain1/1, Mux/1
  Fcn1/1 -> Gain3/1
  Fcn/1 -> Gain2/1
  Mux/1 -> Fcn1/1, Fcn/1

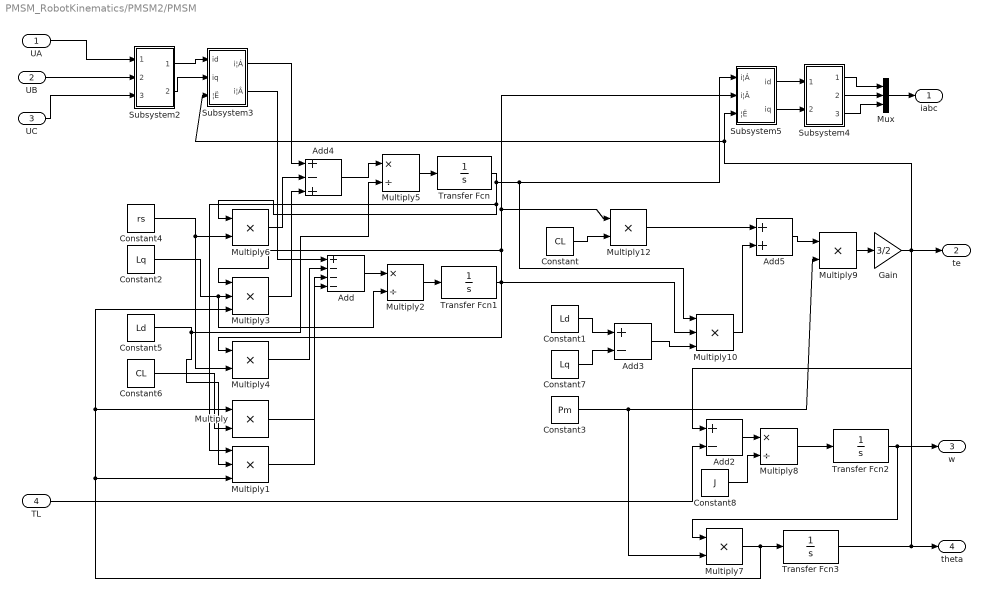
== system PMSM_RobotKinematics/PMSM2/PMSM ==
  UA : Inport
  UB : Inport  Port=2
  UC : Inport  Port=3
  TL : Inport  Port=4
  Add : Sum  Inputs=+---  SaturateOnIntegerOverflow=on  OutDataTypeStr=Inherit: Same as first input
  Add2 : Sum  Inputs=+-  SaturateOnIntegerOverflow=on  InputSameDT=on  OutDataTypeStr=Inherit: Same as first input
  Add3 : Sum  Inputs=+-  SaturateOnIntegerOverflow=on  InputSameDT=on  OutDataTypeStr=Inherit: Same as first input
  Add4 : Sum  Inputs=+-+  SaturateOnIntegerOverflow=on  InputSameDT=on  OutDataTypeStr=Inherit: Same as first input
  Add5 : Sum  SaturateOnIntegerOverflow=on  InputSameDT=on  OutDataTypeStr=Inherit: Same as first input
  Constant : Constant  Value=CL
  Constant1 : Constant  Value=Ld
  Constant2 : Constant  Value=Lq
  Constant3 : Constant  Value=Pm
  Constant4 : Constant  Value=rs
  Constant5 : Constant  Value=Ld
  Constant6 : Constant  Value=CL
  Constant7 : Constant  Value=Lq
  Constant8 : Constant  Value=J
  Gain : Gain  Gain=3/2  SaturateOnIntegerOverflow=on  OutDataTypeStr=Inherit: Same as input  ParamDataTypeStr=Inherit: Same as input
  Multiply{,4,6..7,9,12} (6 alike) : Product  Inputs=**  SaturateOnIntegerOverflow=on  OutDataTypeStr=Inherit: Same as first input
  Multiply1 : Product  Inputs=***  SaturateOnIntegerOverflow=on  OutDataTypeStr=Inherit: Same as first input
  Multiply10 : Product  Inputs=***  SaturateOnIntegerOverflow=on  OutDataTypeStr=Inherit: Same as first input
  Multiply2 : Product  Inputs=*/  SaturateOnIntegerOverflow=on  OutDataTypeStr=Inherit: Same as first input
  Multiply3 : Product  Inputs=***  SaturateOnIntegerOverflow=on  OutDataTypeStr=Inherit: Same as first input
  Multiply5 : Product  Inputs=*/  SaturateOnIntegerOverflow=on  OutDataTypeStr=Inherit: Same as first input
  Multiply8 : Product  Inputs=*/  SaturateOnIntegerOverflow=on  OutDataTypeStr=Inherit: Same as first input
  Mux : Mux  Inputs=3
  Subsystem2 : Subsystem  mask(hao){}
      mask help: 3/2
      mask Help: no
      mask Display: disp('3/2')
  Subsystem3 : Subsystem  mask(2/2){}
      mask help: qdtoMT
      mask Help: none
  Subsystem4 : Subsystem  mask(hao){}
      mask help: 2/3
      mask Help: npi
      mask Display: disp('2/3')
  Subsystem5 : Subsystem  mask(2/2){}
      mask help: mt-todq
      mask Help: no
  Transfer Fcn : TransferFcn  Denominator=[1 0]  AbsoluteTolerance=1e-3
  Transfer Fcn1 : TransferFcn  Denominator=[1 0]
  Transfer Fcn2 : TransferFcn  Denominator=[1 0]
  Transfer Fcn3 : TransferFcn  Denominator=[1 0]
  iabc : Outport
  te : Outport  Port=2
  w : Outport  Port=3
  theta : Outport  Port=4
  wires:
  UB/1 -> Subsystem2/2(In2)
  UA/1 -> Subsystem2/1(In1)
  Subsystem4/2(Out2) -> Mux/2
  Subsystem4/1(Out1) -> Mux/1
  Gain/1 -> Add2/1, te/1
  Transfer Fcn3/1 -> theta/1, Subsystem3/3(¦Ë), Subsystem5/3(¦Ë)
  UC/1 -> Subsystem2/3(In3)
  Multiply8/1 -> Transfer Fcn2/1
  Mux/1 -> iabc/1
  Subsystem4/3(Out3) -> Mux/3
  Multiply9/1 -> Gain/1
  Add5/1 -> Multiply9/1
  Transfer Fcn2/1 -> w/1, Multiply7/1
  Add3/1 -> Multiply10/3
  Constant/1 -> Multiply12/2
  Multiply7/1 -> Multiply1/3, Multiply/1, Multiply3/3, Transfer Fcn3/1
  Constant6/1 -> Multiply/2
  Constant5/1 -> Multiply5/2, Multiply1/2
  Constant2/1 -> Multiply2/2, Multiply3/2
  Transfer Fcn1/1 -> Multiply10/2, Multiply4/1, Subsystem5/2(i¦Â), Multiply12/1, Multiply3/1
  Constant4/1 -> Multiply4/2, Multiply6/2
  Transfer Fcn/1 -> Subsystem5/1(i¦Á), Multiply10/1, Multiply1/1, Multiply6/1
  Subsystem2/1(Out1) -> Subsystem3/1(id)
  Subsystem2/2(Out2) -> Subsystem3/2(iq)
  Subsystem3/1(i¦Á) -> Add4/1
  Multiply6/1 -> Add4/2
  Multiply3/1 -> Add4/3
  Add4/1 -> Multiply5/1
  Subsystem3/2(i¦Â) -> Add/1
  Add/1 -> Multiply2/1
  Multiply4/1 -> Add/2
  Multiply/1 -> Add/3
  Multiply1/1 -> Add/4
  Constant1/1 -> Add3/1
  Constant7/1 -> Add3/2
  Multiply12/1 -> Add5/1
  Multiply10/1 -> Add5/2
  Constant3/1 -> Multiply9/2, Multiply7/2
  Subsystem5/1(id) -> Subsystem4/1(In1)
  Subsystem5/2(iq) -> Subsystem4/2(In3)
  Add2/1 -> Multiply8/1
  Constant8/1 -> Multiply8/2
  TL/1 -> Add2/2
  Multiply5/1 -> Transfer Fcn/1
  Multiply2/1 -> Transfer Fcn1/1

== system PMSM_RobotKinematics/PMSM2/Park ==
  I_alpha : Inport
  I_beta : Inport  Port=2
  Theta : Inport  Port=3
  Fcn : Fcn  Expr=sin(u)
  Fcn1 : Fcn  Expr=cos(u)
  Gain : Gain  SaturateOnIntegerOverflow=on  OutDataTypeStr=Inherit: Same as input  ParamDataTypeStr=Inherit: Same as input
  Gain1 : Gain  SaturateOnIntegerOverflow=on  OutDataTypeStr=Inherit: Same as input  ParamDataTypeStr=Inherit: Same as input
  Mux : Mux  Inputs=[1 1 1 1]
  id : Fcn  Expr=u[1]*u[3]+u[2]*u[4]
  iq : Fcn  Expr=-u[2]*u[3]+u[1]*u[4]
  Id : Outport  InitialOutput=0
  Iq : Outport  Port=2  InitialOutput=0
  wires:
  I_beta/1 -> Mux/4
  Gain1/1 -> Iq/1
  Gain/1 -> Id/1
  id/1 -> Gain/1
  iq/1 -> Gain1/1
  I_alpha/1 -> Mux/3
  Mux/1 -> id/1, iq/1
  Theta/1 -> Fcn/1, Fcn1/1
  Fcn1/1 -> Mux/1
  Fcn/1 -> Mux/2

== system PMSM_RobotKinematics/PMSM2/Park_inv ==
  iq : Inport
  id : Inport  Port=2
  Theta : Inport  Port=3
  Fcn : Fcn  Expr=sin(u)
  Fcn1 : Fcn  Expr=cos(u)
  Gain : Gain  SaturateOnIntegerOverflow=on  OutDataTypeStr=Inherit: Same as input  ParamDataTypeStr=Inherit: Same as input
  Gain1 : Gain  SaturateOnIntegerOverflow=on  OutDataTypeStr=Inherit: Same as input  ParamDataTypeStr=Inherit: Same as input
  Mux : Mux  Inputs=[1 1 1 1]
  i_alpha : Fcn  Expr=u[1]*u[4]-u[2]*u[3]
  i_beta : Fcn  Expr=u[2]*u[4]+u[1]*u[3]
  I_apha : Outport  InitialOutput=0
  I_beta : Outport  Port=2  InitialOutput=0
  wires:
  id/1 -> Mux/4
  Gain1/1 -> I_beta/1
  Gain/1 -> I_apha/1
  i_alpha/1 -> Gain/1
  i_beta/1 -> Gain1/1
  iq/1 -> Mux/3
  Mux/1 -> i_alpha/1, i_beta/1
  Theta/1 -> Fcn/1, Fcn1/1
  Fcn1/1 -> Mux/1
  Fcn/1 -> Mux/2

== system PMSM_RobotKinematics/PMSM2/iqref ==
  In_1 : Inport
  Integral : TransferFcn  Numerator=[I]  Denominator=[1 0]
  Proportional : Gain  Gain=P  SaturateOnIntegerOverflow=on  OutDataTypeStr=Inherit: Same as input  ParamDataTypeStr=Inherit: Same as input
  Saturation : Saturate  UpperLimit=max  LowerLimit=min
  Sum : Sum  SaturateOnIntegerOverflow=on  InputSameDT=on  OutDataTypeStr=Inherit: Same as first input
  Out_1 : Outport  InitialOutput=0
  wires:
  Saturation/1 -> Out_1/1
  Sum/1 -> Saturation/1
  Proportional/1 -> Sum/1
  In_1/1 -> Proportional/1, Integral/1
  Integral/1 -> Sum/2

== system PMSM_RobotKinematics/PMSM2/iqref1 ==
  In_1 : Inport
  Integral : TransferFcn  Numerator=[I]  Denominator=[1 0]
  Proportional : Gain  Gain=P  SaturateOnIntegerOverflow=on  OutDataTypeStr=Inherit: Same as input  ParamDataTypeStr=Inherit: Same as input
  Saturation : Saturate  UpperLimit=max  LowerLimit=min
  Sum : Sum  SaturateOnIntegerOverflow=on  InputSameDT=on  OutDataTypeStr=Inherit: Same as first input
  Out_1 : Outport  InitialOutput=0
  wires:
  Integral/1 -> Sum/2
  In_1/1 -> Integral/1, Proportional/1
  Proportional/1 -> Sum/1
  Sum/1 -> Saturation/1
  Saturation/1 -> Out_1/1

== system PMSM_RobotKinematics/PMSM2/iqref2 ==
  In_1 : Inport
  Integral : TransferFcn  Numerator=[I]  Denominator=[1 0]
  Proportional : Gain  Gain=P  SaturateOnIntegerOverflow=on  OutDataTypeStr=Inherit: Same as input  ParamDataTypeStr=Inherit: Same as input
  Saturation : Saturate  UpperLimit=max  LowerLimit=min
  Sum : Sum  SaturateOnIntegerOverflow=on  InputSameDT=on  OutDataTypeStr=Inherit: Same as first input
  Out_1 : Outport  InitialOutput=0
  wires:
  Integral/1 -> Sum/2
  In_1/1 -> Integral/1, Proportional/1
  Proportional/1 -> Sum/1
  Sum/1 -> Saturation/1
  Saturation/1 -> Out_1/1

== system PMSM_RobotKinematics/PMSM2/iqref3 ==
  In_1 : Inport
  Integral : TransferFcn  Numerator=[I]  Denominator=[1 0]
  Proportional : Gain  Gain=P  SaturateOnIntegerOverflow=on  OutDataTypeStr=Inherit: Same as input  ParamDataTypeStr=Inherit: Same as input
  Saturation : Saturate  UpperLimit=max  LowerLimit=min
  Sum : Sum  SaturateOnIntegerOverflow=on  InputSameDT=on  OutDataTypeStr=Inherit: Same as first input
  Out_1 : Outport  InitialOutput=0
  wires:
  Saturation/1 -> Out_1/1
  Sum/1 -> Saturation/1
  Proportional/1 -> Sum/1
  In_1/1 -> Proportional/1, Integral/1
  Integral/1 -> Sum/2

== system PMSM_RobotKinematics/PMSM3/Clarke ==
  is_abc : Inport
  Gain : Gain  Gain=sqrt(3/2)  SaturateOnIntegerOverflow=on  OutDataTypeStr=Inherit: Same as input  ParamDataTypeStr=Inherit: Same as input
  Gain1 : Gain  Gain=sqrt(2)/2  SaturateOnIntegerOverflow=on  OutDataTypeStr=Inherit: Same as input  ParamDataTypeStr=Inherit: Same as input
  Mux : Mux  Inputs=[3]
  i_alpha : Fcn  Expr=u[1]
  i_beta : Fcn  Expr=u[1]+2*u[2]
  I_alpha : Outport  InitialOutput=0
  I_beta : Outport  Port=2  InitialOutput=0
  wires:
  Mux/1 -> i_beta/1, i_alpha/1
  is_abc/1 -> Mux/1
  i_beta/1 -> Gain1/1
  i_alpha/1 -> Gain/1
  Gain/1 -> I_alpha/1
  Gain1/1 -> I_beta/1

== system PMSM_RobotKinematics/PMSM3/Clarke_inv ==
  Valpha : Inport
  Vbeta : Inport  Port=2
  Fcn : Fcn  Expr=-u[1]/2+1.73205081*u[2]/2
  Fcn1 : Fcn  Expr=-u[1]/2-1.73205081*u[2]/2
  Gain1 : Gain  Gain=sqrt(2/3)  SaturateOnIntegerOverflow=on  OutDataTypeStr=Inherit: Same as input  ParamDataTypeStr=Inherit: Same as input
  Gain2 : Gain  Gain=sqrt(2/3)  SaturateOnIntegerOverflow=on  OutDataTypeStr=Inherit: Same as input  ParamDataTypeStr=Inherit: Same as input
  Gain3 : Gain  Gain=sqrt(2/3)  SaturateOnIntegerOverflow=on  OutDataTypeStr=Inherit: Same as input  ParamDataTypeStr=Inherit: Same as input
  Mux : Mux  Inputs=2
  Va : Outport
  Vb : Outport  Port=2
  Vc : Outport  Port=3
  wires:
  Mux/1 -> Fcn/1, Fcn1/1
  Fcn/1 -> Gain2/1
  Fcn1/1 -> Gain3/1
  Valpha/1 -> Mux/1, Gain1/1
  Vbeta/1 -> Mux/2
  Gain1/1 -> Va/1
  Gain2/1 -> Vb/1
  Gain3/1 -> Vc/1
